simulink model "scon2_L8_1ponto1_simulink"  (R2024a)
settings: Solver=ode4  StartTime=0.0  StopTime=10.0  RelTol=1e-3
values from neighbouring files (symbols this model uses):
  A = [0, 1, 0; 0, 0, 1; 0, -4, -5]    [scon2_L8_1ponto1.m]
  B = [0; 0; 1]    [scon2_L8_1ponto1.m]
  C = [4, 0, 0]    [scon2_L8_1ponto1.m]
  K = acker(A,B,J)    [scon2_L8_1ponto1.m]
  th_ref = 5*2*pi    (= 31.4159265359)    [scon2_L8_1ponto1.m]
settings Model: Creator=NIA  LastModifiedBy=Carlos Augusto
settings ModelReferenceCC: EnableRefExpFcnMdlSchedulingChecks=on
settings RTWCC: GPUComputeCapability=3.5

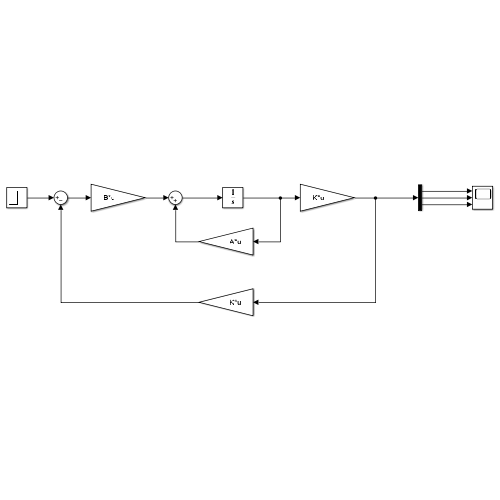
[thumbnail: Simulink's stored preview of the top-level diagram]
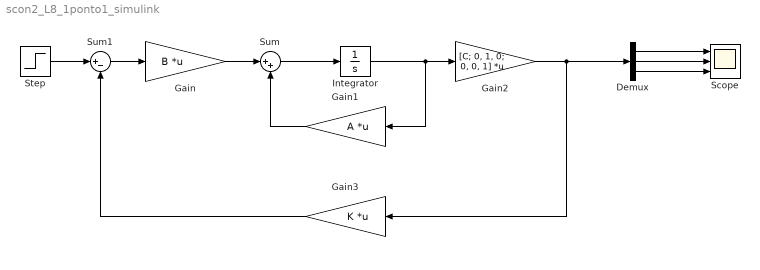
== system scon2_L8_1ponto1_simulink ==
  Demux : Demux  Outputs=3
  Gain : Gain  Gain=B  Multiplication=Matrix(K*u)
  Gain1 : Gain  Gain=A  Multiplication=Matrix(K*u)
  Gain2 : Gain  Gain=[C; 0, 1, 0; 0, 0, 1]  Multiplication=Matrix(K*u)
  Gain3 : Gain  Gain=K  Multiplication=Matrix(K*u)
  Integrator : Integrator
  Scope : Scope  NumInputPorts=3
  Step : Step  After=th_ref  SampleTime=0
  Sum : Sum  Inputs=|++
  Sum1 : Sum  Inputs=|+-
  wires:
  Gain/1 -> Sum/1
  Gain1/1 -> Sum/2
  Sum/1 -> Integrator/1
  Integrator/1 -> Gain2/1, Gain1/1
  Step/1 -> Sum1/1
  Sum1/1 -> Gain/1
  Gain3/1 -> Sum1/2
  Gain2/1 -> Demux/1, Gain3/1
  Demux/1 -> Scope/1
  Demux/2 -> Scope/2
  Demux/3 -> Scope/3
